simulink model "AynchronousEKF_SimpleCircleTrajectory"  (R2025b)
settings: Solver=VariableStepAuto  StartTime=0.0  StopTime=100  RelTol=1e-3
undefined symbols (not defined in the file or in its folder): cam1_sample_time, cam2_sample_time, cam3_sample_time, cam_intrinsics, dt_ekf, focusLength_narrow, gray, num_cams, omega, pixelSize, radius, Rec, resolution, SDTV, Sim3dSensor, waypointTrajectory
libraries: sim3dlib x10, robotcorelib x7, visionconversions x6, sim3dcameralib x3, uavutilslib x1, uavsim3dlib x1, uavalgslib x1, dspnetwork x1
settings Model: Creator=nnekoo  LastModifiedBy=Shannon Pitman

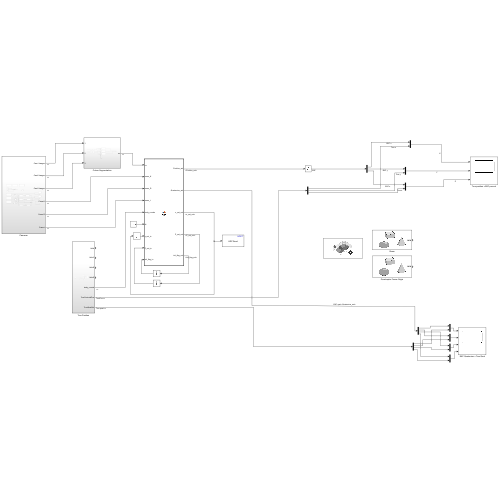
[thumbnail: Simulink's stored preview of the top-level diagram]
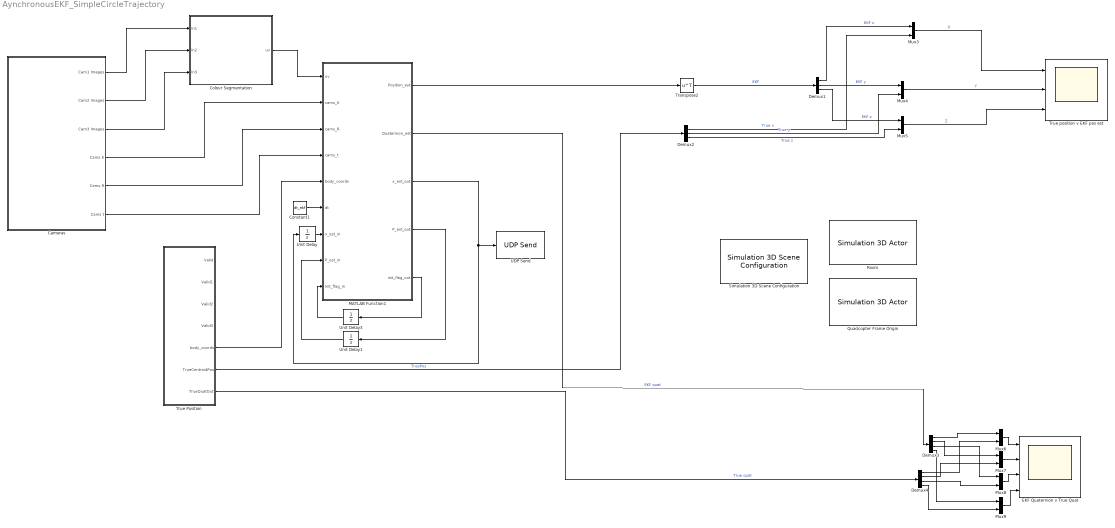
== system AynchronousEKF_SimpleCircleTrajectory ==
  " EKF Quaternion v True Quat" : Scope  NumInputPorts=4
      settings: ActiveDisplayYMinimum=-1.2499889931974075  ActiveDisplayYMaximum=1.2499985502233475  DataLoggingVariableName=ScopeData2
  Cameras : Subsystem
  Colour Segmentation : Subsystem
  Constant1 : Constant  Value=dt_ekf
  Demux1 : Demux  Outputs=3
  Demux2 : Demux  Outputs=3
  Demux3 : Demux
  Demux4 : Demux
  MATLAB Function1 : MATLAB Function  TreatAsAtomicUnit=on
  Mux{3..9} (7 alike) : Mux  Inputs=2
  Quadcopter Frame Origin : sim3dlib/Simulation 3D Actor  Priority=1  ActorName=QuadcopterOrigin  ParentName=Quadcopter  Operation=Create at setup  InitScriptText=|  SampleTime=-1  Translation=[0 0 0]  Rotation=[0 0 0]  Scale=[.01 .01 .01]  aMode=aMode  ActorTag=QuadcopterOrigin  ActorType=Sim3dActor  ID=C
      | createShape(Actor, 'cylinder', [1 1 1]);
      | 
      | Actor.Color = [255 192 203]/255;
      | Actor.Mobility = sim3d.utils.MobilityTypes.Movable;
  Room : sim3dlib/Simulation 3D Actor  Priority=1  ActorName=Room  ParentName=Scene Origin  Operation=Create at setup  InitScriptText=|  SampleTime=-1  Translation=[0 0 0]  Rotation=[0 0 0]  Scale=[1 1 1]  aMode=5  ActorTag=Room  ActorType=Sim3dActor  ID=C
      | leftWall = sim3d.Actor(ActorName="leftWall");
      | createShape(leftWall, 'plane', [8 5 1]);
      | leftWall.Rotation = [pi/2 0 0];
      | leftWall.Translation = [0 -4.5 1.5];
      | leftWall.Color = [1 1 1];
      | World.add(leftWall,Actor);
      | 
      | rightWall = sim3d.Actor(ActorName="rightWall");
      | createShape(rightWall, 'plane', [8 5 1]);
      | % rightWall.CoordinateSystem = 'MATLAB';
      | rightWall.Rotation = [pi/2 0 0];
      | rightWall.Translation = [0 4.5 1.5];
      | rightWall.Color = [1 1 1];
      | World.add(rightWall,Actor);
      | 
      | farWall = sim3d.Actor(ActorName="farWall");
      | createShape(farWall, 'plane', [9 5 1]);
      | % farWall.CoordinateSystem = 'MATLAB';
      | farWall.Rotation = [pi/2 0 pi/2];
      | farWall.Translation = [4 0 1.5];
      | farWall.TwoSided = true;
      | farWall.Color = [1 1 1];
      | World.add(farWall,Actor);
      | 
      | floor = sim3d.Actor(ActorName="floor");
      | createShape(floor, 'plane', [8 9 .5]);
      | % floor.CoordinateSystem = 'MATLAB';
      | floor.Translation = [0 0 -1];
      | floor.Rotation = [0 0 0];
      | floor.Color = [1 1 1];
      | World.add(floor,Actor);
      | 
      | ceiling = sim3d.Actor(ActorName="ceiling");
      | createShape(ceiling, 'plane', [8 9 .5]);
      | % floor.CoordinateSystem = 'MATLAB';
      | ceiling.Translation = [0 0 4];
      | ceiling.Rotation = [0 0 0];
      | ceiling.Color = [1 1 1];
      | World.add(ceiling,Actor);
      | 
      | frontWall = sim3d.Actor(ActorName="frontWall");
      | createShape(frontWall, 'plane', [9 5 1]);
      | % floor.CoordinateSystem = 'MATLAB';
      | frontWall.Rotation = [pi/2 0 pi/2];
      | frontWall.Translation = [-4 0 1.5];
      | World.add(frontWall,Actor);
      | 
      | lights = sim3d.Light(ActorName = 'ceilingLights', NumberOfLights=7, LightType = 'PointLight', Translation = [-3 -3 3.9; 3 -3 3.9;0 -3 3.9; 0 3 3.9; -3 3 3.9;3 3 3.9; 0 0 3.9 ]);
      | World.add(lights, Actor);
      | %, Rotation = [pi/2 0 pi/2; pi/2 0 pi/2; pi/2 0 pi/2; pi/2 0 pi/2]
  Simulation 3D Scene Configuration : sim3dlib/Simulation 3D Scene Configuration  Priority=0  ProjectFormat=Default Scenes  SceneDesc=Empty scene  ProjectName=C:\Program Files\MATLAB\R2025b\toolbox\shared\sim3d_projects\automotive_project_windows\UE\WindowsNoEditor\VehicleSimulation.exe  ScenePath=/Game/Maps/HwStrght  UEProjPath=C:\project\AutoVrtlEnv\AutoVrtlEnv.uproject  EnableOpenDRIVE=off  vehTagList={'Cam1';'Cam2';'Cam3';'Custom';'FrontLeftMotor';'FrontRightMotor';'Quadcopter';'QuadcopterOrigin';'RearLeftMotor';'RearRightMotor';'Room';'Scene Origin'}  vehTag=Custom  AttachedCameraRelativeTranslation=[0 0 0]  FreeCameraDefaultInitialTranslation=[-6, 0, 2]  AttachedCameraRelativeRotation=[0 0 0]  FreeCameraDefaultInitialRotation=[0, -15, 0]  ViewpointName=Custom  FreeCameraInitialTranslation=[-3 0 0.5]  ViewpointTranslation=[0 0 0]  FreeCameraInitialRotation=[0 -10 0]  ViewpointRotation=[0 0 0]  OpVisEn=off  Ts=1/60  EnableWindow=off  EnableRemoteAccess=off  EnableWeather=off  SunAzimuth=90  SunAltitude=40.0  EnableGeospatialSun=off  Latitude=0  Longitude=0  Date=2023-01-01  Time=10:30:00  GeoTimeZone=-5.0  SunDaylightSaving=off  wind=1  clouds=10  EnableVolumetricClouds=off  CloudCoverage=0  CloudAltitude=6  fog=0  rain=0  RaindropsEffect=off  SnowDensity=0  EnableGeospatial=off  TilesetSource=Earth terrain  UseTrueOrigin=off  OriginHeight=200  OriginLatitude=40.744652  OriginLongitude=-73.988864  MapStyle=Aerial  AdditionalAssetIDs=[]  UseAdvancedSunSky=off  SolarTime=11  TimeZone=-5  Day=21  Month=9  Year=2022  UseDaylightSavingTime=on  DSTStartDay=10  DSTStartMonth=3  DSTEndDay=3  DSTEndMonth=11  DSTSwitchHour=2  sensorTag=MainCamera1  sensorId=1  sensorName=MainCamera1  mountLoc=Origin  offsetFlag=off  tmountOffset=[0, 0, 0]  rmountOffset=[0, 0, 0]  HorizontalResolution=1280  VerticalResolution=720  HorizontalFOV=60  mountPoint=[0 0 0]  mountOrientation=[0 0 0]  aMode=5  ID=1  GeoTrigger=Inactive  ViewNameList={'Custom'}  ViewTranslationList={'[-3 0 0.5]'}  ViewRotationList={'[0 -10 0]'}
      settings: LibrarySourceBlock=sl3dlib/Simulation 3D/Environment/Simulation 3D Scene Configuration
  Transpose2 : Math  Operator=transpose
  True Position : Subsystem
  True position v EKF pos est : Scope  NumInputPorts=3
      settings: ActiveDisplayYMinimum=1.2433440169653658  ActiveDisplayYMaximum=2.8099234426996063
  UDP Send : dspnetwork/UDP Send  remoteURL='127.0.0.1'  remotePort=25000  localURL='0.0.0.0'  localPortSource=Automatically determine  localPort=-1  sendBufferSize=8192  sampletime=-1  blockPlatform=HOST  separateLengthPort=0
      settings: LibrarySourceBlock=embeddedtargetslib/Host Communication/UDP Send
  Unit Delay : UnitDelay  InitialCondition=zeros(13,1)  SampleTime=dt_ekf  StateName=Previous State Estimate  HasFrameUpgradeWarning=on
  Unit Delay1 : UnitDelay  InitialCondition=zeros(13,13)  SampleTime=dt_ekf  StateName=Previous State Error Covariance Estimate  HasFrameUpgradeWarning=on
  Unit Delay3 : UnitDelay  SampleTime=dt_ekf  StateName=EKF has been initialised  HasFrameUpgradeWarning=on
  wires:
  MATLAB Function1/1(Position_est) -> Transpose2/1
  Constant1/1 -> MATLAB Function1/6(dt)
  True Position/5(body_coords) -> MATLAB Function1/5(body_coords)
  MATLAB Function1/2(Quaternion_est) -> Demux3/1  "EKF quat"
  MATLAB Function1/3(x_est_out) -> UDP Send/1, Unit Delay/1
  Unit Delay/1 -> MATLAB Function1/7(x_est_in)
  Unit Delay1/1 -> MATLAB Function1/8(P_est_in)
  Unit Delay3/1 -> MATLAB Function1/9(init_flag_in)
  Transpose2/1 -> Demux1/1  "EKF"
  Demux1/1 -> Mux3/1  "EKF x"
  Demux2/1 -> Mux3/2  "True x"
  Demux1/2 -> Mux4/1  "EKF y"
  Demux2/2 -> Mux4/2  "True y"
  Demux1/3 -> Mux5/1  "EKF z"
  Mux3/1 -> True position v EKF pos est/1  "X"
  Demux2/3 -> Mux5/2  "True z"
  Mux4/1 -> True position v EKF pos est/2  "Y"
  Mux5/1 -> True position v EKF pos est/3  "Z"
  Demux3/1 -> Mux6/1
  Demux4/1 -> Mux6/2
  Mux6/1 -> " EKF Quaternion v True Quat"/1
  Demux3/2 -> Mux7/1
  Demux4/2 -> Mux7/2
  Mux7/1 -> " EKF Quaternion v True Quat"/2
  Demux3/3 -> Mux8/1
  Demux4/3 -> Mux8/2
  Mux8/1 -> " EKF Quaternion v True Quat"/3
  Demux3/4 -> Mux9/1
  Demux4/4 -> Mux9/2
  Mux9/1 -> " EKF Quaternion v True Quat"/4
  True Position/6(TrueCentroidPos) -> Demux2/1  "TruePos"
  True Position/7(TrueQuatOut) -> Demux4/1  "True quat"
  Cameras/1(Cam1 Images) -> Colour Segmentation/1(In1)
  Cameras/2(Cam2 Images) -> Colour Segmentation/2(In2)
  Cameras/3(Cam3 Images) -> Colour Segmentation/3(In3)
  Cameras/4(Cams.K) -> MATLAB Function1/2(cams_K)
  Cameras/5(Cams.R) -> MATLAB Function1/3(cams_R)
  Cameras/6(Cams.t) -> MATLAB Function1/4(cams_t)
  Colour Segmentation/1(uv) -> MATLAB Function1/1(uv)
  MATLAB Function1/5(init_flag_out) -> Unit Delay3/1
  MATLAB Function1/4(P_est_out) -> Unit Delay1/1

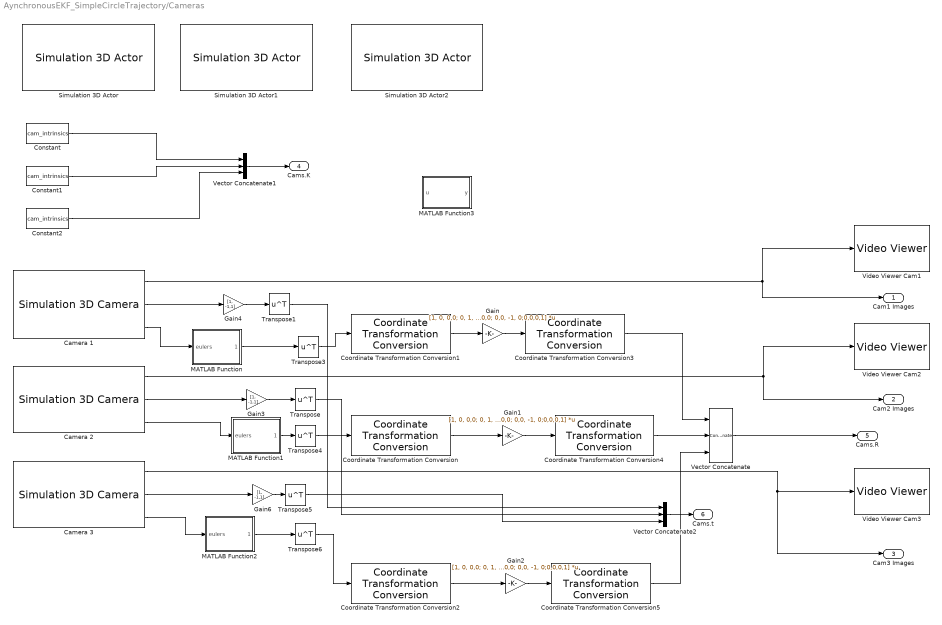
== system AynchronousEKF_SimpleCircleTrajectory/Cameras ==
  Camera 1 : sim3dcameralib/Simulation 3D Camera  Priority=1  sensorTag=Sim3dSensor�  sensorId=1  sensorName=Sim3dSensor�  vehTagList={'Cam1';'Cam2';'Cam3';'FrontLeftMotor';'FrontRightMotor';'Quadcopter';'QuadcopterOrigin';'RearLeftMotor';'RearRightMotor';'Room';'Scene Origin'}  vehTag=Scene Origin  CoordinateSystem=Default  mountLoc=Origin  offsetFlag=on  tmountOffset=[0, -2, 0.5]  extTmount=off  rmountOffset=[0, 0, pi/4]  extRmount=off  FocalLength=[focusLength_narrow/pixelSize(1), focusLength_narrow/pixelSize(2)]  OpticalCenter=[resolution(2)/2 resolution(1)/2]  ImageSize=resolution  RadialDistortion=[0, 0]  TangentialDistortion=[0, 0]  SensorSkew=0  VisualizeFieldOfView=off  FieldOfViewRange=61  DepthOutportEnabled=off  SemanticOutportEnabled=off  TransformOutportEnabled=on  SampleTime=cam1_sample_time  mountPoint=[0 -2 0.5]  mountOrientation=[0 0 0.785398163397448]  aMode=5  ID=1
      settings: LibrarySourceBlock=sl3dlib/Simulation 3D/Sensors/Simulation 3D Camera
  Camera 2 : sim3dcameralib/Simulation 3D Camera  Priority=1  sensorTag=Sim3dSensor�  sensorId=2  sensorName=Sim3dSensor�  vehTagList={'Cam1';'Cam2';'Cam3';'FrontLeftMotor';'FrontRightMotor';'Quadcopter';'QuadcopterOrigin';'RearLeftMotor';'RearRightMotor';'Room';'Scene Origin'}  vehTag=Scene Origin  CoordinateSystem=Default  mountLoc=Origin  offsetFlag=on  tmountOffset=[0, 2, 0.5]  extTmount=off  rmountOffset=[0, 0, -pi/4]  extRmount=off  FocalLength=[focusLength_narrow/pixelSize(1), focusLength_narrow/pixelSize(2)]  OpticalCenter=[resolution(2)/2 resolution(1)/2]  ImageSize=resolution  RadialDistortion=[0, 0]  TangentialDistortion=[0, 0]  SensorSkew=0  VisualizeFieldOfView=off  FieldOfViewRange=61  DepthOutportEnabled=off  SemanticOutportEnabled=off  TransformOutportEnabled=on  SampleTime=cam2_sample_time  mountPoint=[0 2 0.5]  mountOrientation=[0 0 -0.785398163397448]  aMode=5  ID=2
      settings: LibrarySourceBlock=sl3dlib/Simulation 3D/Sensors/Simulation 3D Camera
  Camera 3 : sim3dcameralib/Simulation 3D Camera  Priority=1  sensorTag=Sim3dSensor�  sensorId=3  sensorName=Sim3dSensor�  vehTagList={'Cam1';'Cam2';'Cam3';'FrontLeftMotor';'FrontRightMotor';'Quadcopter';'QuadcopterOrigin';'RearLeftMotor';'RearRightMotor';'Room';'Scene Origin'}  vehTag=Scene Origin  CoordinateSystem=Default  mountLoc=Origin  offsetFlag=on  tmountOffset=[2.5,-1.5,0.5]  extTmount=off  rmountOffset=[0, 0, pi/2]  extRmount=off  FocalLength=[focusLength_narrow/pixelSize(1), focusLength_narrow/pixelSize(2)]  OpticalCenter=[resolution(2)/2 resolution(1)/2]  ImageSize=resolution  RadialDistortion=[0, 0]  TangentialDistortion=[0, 0]  SensorSkew=0  VisualizeFieldOfView=off  FieldOfViewRange=61  DepthOutportEnabled=off  SemanticOutportEnabled=off  TransformOutportEnabled=on  SampleTime=cam3_sample_time  mountPoint=[2.5 -1.5 0.5]  mountOrientation=[0 0 1.5707963267949]  aMode=5  ID=3
      settings: LibrarySourceBlock=sl3dlib/Simulation 3D/Sensors/Simulation 3D Camera
  Constant : Constant  Value=cam_intrinsics  VectorParams1D=off
  Constant1 : Constant  Value=cam_intrinsics  VectorParams1D=off
  Constant2 : Constant  Value=cam_intrinsics  VectorParams1D=off
  Coordinate Transformation Conversion : robotcorelib/Coordinate Transformation Conversion  InputRepresentation=Euler Angles  InputEulerSequence=ZYX  ShowTrVecInputPort=on  OutputRepresentation=Quaternion  OutputEulerSequence=ZYX  ShowTrVecOutputPort=on  SimulateUsing=Interpreted execution
      settings: LibrarySourceBlock=navlib/Utilities/Coordinate Transformation Conversion
  Coordinate Transformation Conversion1 : robotcorelib/Coordinate Transformation Conversion  InputRepresentation=Euler Angles  InputEulerSequence=ZYX  ShowTrVecInputPort=on  OutputRepresentation=Quaternion  OutputEulerSequence=ZYX  ShowTrVecOutputPort=on  SimulateUsing=Interpreted execution
      settings: LibrarySourceBlock=navlib/Utilities/Coordinate Transformation Conversion
  Coordinate Transformation Conversion2 : robotcorelib/Coordinate Transformation Conversion  InputRepresentation=Euler Angles  InputEulerSequence=ZYX  ShowTrVecInputPort=on  OutputRepresentation=Quaternion  OutputEulerSequence=ZYX  ShowTrVecOutputPort=on  SimulateUsing=Interpreted execution
      settings: LibrarySourceBlock=navlib/Utilities/Coordinate Transformation Conversion
  Coordinate Transformation Conversion3 : robotcorelib/Coordinate Transformation Conversion  InputRepresentation=Quaternion  InputEulerSequence=XYZ  ShowTrVecInputPort=on  OutputRepresentation=Rotation Matrix  OutputEulerSequence=ZYX  ShowTrVecOutputPort=on  SimulateUsing=Interpreted execution
      settings: LibrarySourceBlock=navlib/Utilities/Coordinate Transformation Conversion
  Coordinate Transformation Conversion4 : robotcorelib/Coordinate Transformation Conversion  InputRepresentation=Quaternion  InputEulerSequence=XYZ  ShowTrVecInputPort=on  OutputRepresentation=Rotation Matrix  OutputEulerSequence=ZYX  ShowTrVecOutputPort=on  SimulateUsing=Interpreted execution
      settings: LibrarySourceBlock=navlib/Utilities/Coordinate Transformation Conversion
  Coordinate Transformation Conversion5 : robotcorelib/Coordinate Transformation Conversion  InputRepresentation=Quaternion  InputEulerSequence=XYZ  ShowTrVecInputPort=on  OutputRepresentation=Rotation Matrix  OutputEulerSequence=ZYX  ShowTrVecOutputPort=on  SimulateUsing=Interpreted execution
      settings: LibrarySourceBlock=navlib/Utilities/Coordinate Transformation Conversion
  Gain : Gain  Gain=[1, 0, 0,0; 0, 1, 0,0; 0,0, -1, 0;0,0,0,1]  Multiplication=Matrix(K*u)
  Gain1 : Gain  Gain=[1, 0, 0,0; 0, 1, 0,0; 0,0, -1, 0;0,0,0,1]  Multiplication=Matrix(K*u)
  Gain2 : Gain  Gain=[1, 0, 0,0; 0, 1, 0,0; 0,0, -1, 0;0,0,0,1]  Multiplication=Matrix(K*u)
  Gain3 : Gain  Gain=[1, -1,1]
  Gain4 : Gain  Gain=[1, -1,1]
  Gain6 : Gain  Gain=[1, -1,1]
  MATLAB Function : MATLAB Function  TreatAsAtomicUnit=on
  MATLAB Function1 : MATLAB Function  TreatAsAtomicUnit=on
  MATLAB Function2 : MATLAB Function  TreatAsAtomicUnit=on
  MATLAB Function3 : MATLAB Function  TreatAsAtomicUnit=on
  Simulation 3D Actor : sim3dlib/Simulation 3D Actor  Priority=1  ActorName=Cam1  ParentName=Camera1  Operation=Create at setup  InitScriptText=|  SampleTime=-1  Translation=[0 0 0]  Rotation=[0 0 0]  Scale=[1 1 1]  aMode=5  ActorTag=Cam1  ActorType=Sim3dActor  ID=C
      | createShape(Actor, 'cylinder', [0.1 0.1 0.1]);
      | 
      | % Initialize values (optional)
      | Actor.Color = [0 0 0];
      | Actor.CoordinateSystem = 'MATLAB';
      | 
      | % Reserved keywords:
      | % - Actor : handle to this actor object
      | % - World : handle to the world object
      | 
      | % Examples:
      | 
      | % Create a primitive geometry (optional)
      | % createShape(Actor, 'box', [1 1 1]);
      | 
      | % Initialize values (optional)
      | % Actor.Physics = true;
      | % Actor.Color = [1 0 0];
  Simulation 3D Actor1 : sim3dlib/Simulation 3D Actor  Priority=1  ActorName=Cam2  ParentName=Camera2  Operation=Create at setup  InitScriptText=|  SampleTime=-1  Translation=[0 0 0]  Rotation=[0 0 0]  Scale=[1 1 1]  aMode=5  ActorTag=Cam2  ActorType=Sim3dActor  ID=C
      | createShape(Actor, 'cylinder', [0.1 0.1 0.1]);
      | 
      | % Initialize values (optional)
      | Actor.Color = [1 0.65 0];
      | Actor.CoordinateSystem = 'MATLAB';
      | % Reserved keywords:
      | % - Actor : handle to this actor object
      | % - World : handle to the world object
      | 
      | % Examples:
      | 
      | % Create a primitive geometry (optional)
      | % createShape(Actor, 'box', [1 1 1]);
      | 
      | % Initialize values (optional)
      | % Actor.Physics = true;
      | % Actor.Color = [1 0 0];
  Simulation 3D Actor2 : sim3dlib/Simulation 3D Actor  Priority=1  ActorName=Cam3  ParentName=Camera3  Operation=Create at setup  InitScriptText=|  SampleTime=-1  Translation=[0 0 0]  Rotation=[0 0 0]  Scale=[1 1 1]  aMode=5  ActorTag=Cam3  ActorType=Sim3dActor  ID=C
      | createShape(Actor, 'cylinder', [0.1 0.1 0.1]);
      | 
      | % Initialize values (optional)
      | Actor.Color = [1 1 1];
      | Actor.CoordinateSystem = 'MATLAB';
      | % Reserved keywords:
      | % - Actor : handle to this actor object
      | % - World : handle to the world object
      | 
      | % Examples:
      | 
      | % Create a primitive geometry (optional)
      | % createShape(Actor, 'box', [1 1 1]);
      | 
      | % Initialize values (optional)
      | % Actor.Physics = true;
      | % Actor.Color = [1 0 0];
  Transpose{,1,3..6} (6 alike) : Math  Operator=transpose
  Vector Concatenate : Concatenate  NumInputs=3  Mode=Multidimensional array
  Vector Concatenate1 : Concatenate  NumInputs=3  Mode=Multidimensional array
  Vector Concatenate2 : Concatenate  NumInputs=3
  Video Viewer Cam1 : VideoViewer  colormapValue=gray(256)  FigPos=[-793 733 418 262]
  Video Viewer Cam2 : VideoViewer  colormapValue=gray(256)  FigPos=[-1221 623 418 282]
  Video Viewer Cam3 : VideoViewer  colormapValue=gray(256)  FigPos=[-1491 936 417 301]
  Cam1 Images : Outport
  Cam2 Images : Outport  Port=2
  Cam3 Images : Outport  Port=3
  Cams.K : Outport  Port=4
  Cams.R : Outport  Port=5
  Cams.t : Outport  Port=6
  wires:
  Transpose3/1 -> Coordinate Transformation Conversion1/1
  Transpose6/1 -> Coordinate Transformation Conversion2/1
  Transpose4/1 -> Coordinate Transformation Conversion/1
  Constant/1 -> Vector Concatenate1/1
  Constant1/1 -> Vector Concatenate1/2
  Constant2/1 -> Vector Concatenate1/3
  Vector Concatenate/1 -> Cams.R/1
  Vector Concatenate1/1 -> Cams.K/1
  Vector Concatenate2/1 -> Cams.t/1
  Camera 3/2 -> Gain6/1
  Camera 2/2 -> Gain3/1
  Camera 1/2 -> Gain4/1
  Coordinate Transformation Conversion1/1 -> Gain/1
  Coordinate Transformation Conversion/1 -> Gain1/1
  Coordinate Transformation Conversion2/1 -> Gain2/1
  Transpose1/1 -> Vector Concatenate2/1
  Transpose/1 -> Vector Concatenate2/2
  Transpose5/1 -> Vector Concatenate2/3
  Gain6/1 -> Transpose5/1
  Gain3/1 -> Transpose/1
  Gain4/1 -> Transpose1/1
  Camera 2/3 -> MATLAB Function1/1(eulers)
  Camera 3/3 -> MATLAB Function2/1(eulers)
  Camera 1/3 -> MATLAB Function/1(eulers)
  Gain/1 -> Coordinate Transformation Conversion3/1
  Coordinate Transformation Conversion3/1 -> Vector Concatenate/1
  Gain1/1 -> Coordinate Transformation Conversion4/1
  Coordinate Transformation Conversion4/1 -> Vector Concatenate/2
  Gain2/1 -> Coordinate Transformation Conversion5/1
  Coordinate Transformation Conversion5/1 -> Vector Concatenate/3
  MATLAB Function/1(eulerZYX) -> Transpose3/1
  MATLAB Function1/1(eulerZYX) -> Transpose4/1
  MATLAB Function2/1(eulerZYX) -> Transpose6/1
  Camera 1/1 -> Cam1 Images/1, Video Viewer Cam1/1
  Camera 2/1 -> Cam2 Images/1, Video Viewer Cam2/1
  Camera 3/1 -> Cam3 Images/1, Video Viewer Cam3/1

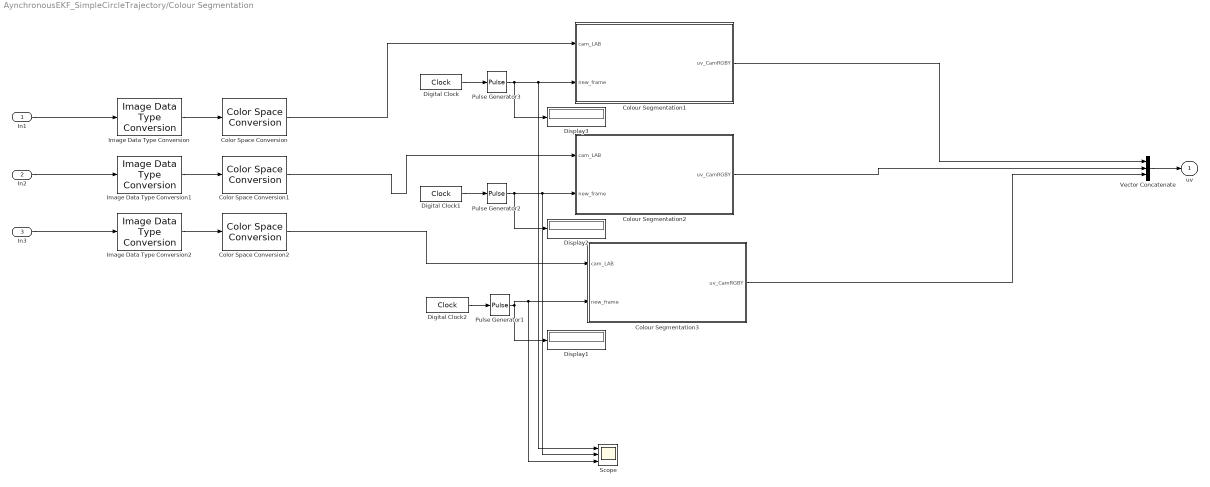
== system AynchronousEKF_SimpleCircleTrajectory/Colour Segmentation ==
  In1 : Inport
  In2 : Inport  Port=2
  In3 : Inport  Port=3
  Color Space Conversion : visionconversions/Color Space  Conversion  conversion=Obsolete  conversionActive=sR'G'B' to L*a*b*  wp_str=D65  rec=Rec. 601 (SDTV)  sys=1125/60/2:1  imagePorts=One multidimensional signal
  Color Space Conversion1 : visionconversions/Color Space  Conversion  conversion=Obsolete  conversionActive=sR'G'B' to L*a*b*  wp_str=D65  rec=Rec. 601 (SDTV)  sys=1125/60/2:1  imagePorts=One multidimensional signal
  Color Space Conversion2 : visionconversions/Color Space  Conversion  conversion=Obsolete  conversionActive=sR'G'B' to L*a*b*  wp_str=D65  rec=Rec. 601 (SDTV)  sys=1125/60/2:1  imagePorts=One multidimensional signal
  Colour Segmentation1 : MATLAB Function  TreatAsAtomicUnit=on
  Colour Segmentation2 : MATLAB Function  TreatAsAtomicUnit=on
  Colour Segmentation3 : MATLAB Function  TreatAsAtomicUnit=on
  Digital Clock : DigitalClock  SampleTime=cam1_sample_time/num_cams
  Digital Clock1 : DigitalClock  SampleTime=cam2_sample_time/num_cams
  Digital Clock2 : DigitalClock  SampleTime=cam3_sample_time/num_cams
  Display1 : Display
  Display2 : Display
  Display3 : Display
  Image Data Type Conversion : visionconversions/Image Data Type Conversion  outDT=double  isSigned=on  wordLen=16  numFracBits=0
  Image Data Type Conversion1 : visionconversions/Image Data Type Conversion  outDT=double  isSigned=on  wordLen=16  numFracBits=0
  Image Data Type Conversion2 : visionconversions/Image Data Type Conversion  outDT=double  isSigned=on  wordLen=16  numFracBits=0
  Pulse Generator1 : DiscretePulseGenerator  TimeSource=Use external signal  Period=3  PhaseDelay=2  SampleTime=1/60
  Pulse Generator2 : DiscretePulseGenerator  TimeSource=Use external signal  Period=3  PhaseDelay=1  SampleTime=1/60
  Pulse Generator3 : DiscretePulseGenerator  TimeSource=Use external signal  Period=3  SampleTime=1/60
  Scope : Scope  NumInputPorts=3
      settings: ActiveDisplayYMinimum=-0.036926070641322362  ActiveDisplayYMaximum=1.1105177004394333
  Vector Concatenate : Concatenate  NumInputs=3  Mode=Multidimensional array
  uv : Outport
  wires:
  Image Data Type Conversion/1 -> Color Space Conversion/1
  Image Data Type Conversion1/1 -> Color Space Conversion1/1
  Colour Segmentation1/1(uv_CamRGBY) -> Vector Concatenate/1
  Colour Segmentation2/1(uv_CamRGBY) -> Vector Concatenate/2
  Color Space Conversion1/1 -> Colour Segmentation2/1(cam_LAB)
  In1/1 -> Image Data Type Conversion/1
  In2/1 -> Image Data Type Conversion1/1
  In3/1 -> Image Data Type Conversion2/1
  Image Data Type Conversion2/1 -> Color Space Conversion2/1
  Vector Concatenate/1 -> uv/1
  Colour Segmentation3/1(uv_CamRGBY) -> Vector Concatenate/3
  Pulse Generator3/1 -> Display3/1, Scope/1, Colour Segmentation1/2(new_frame)
  Color Space Conversion2/1 -> Colour Segmentation3/1(cam_LAB)
  Color Space Conversion/1 -> Colour Segmentation1/1(cam_LAB)
  Digital Clock/1 -> Pulse Generator3/1
  Digital Clock1/1 -> Pulse Generator2/1
  Pulse Generator2/1 -> Scope/2, Colour Segmentation2/2(new_frame), Display2/1
  Digital Clock2/1 -> Pulse Generator1/1
  Pulse Generator1/1 -> Colour Segmentation3/2(new_frame), Scope/3, Display1/1

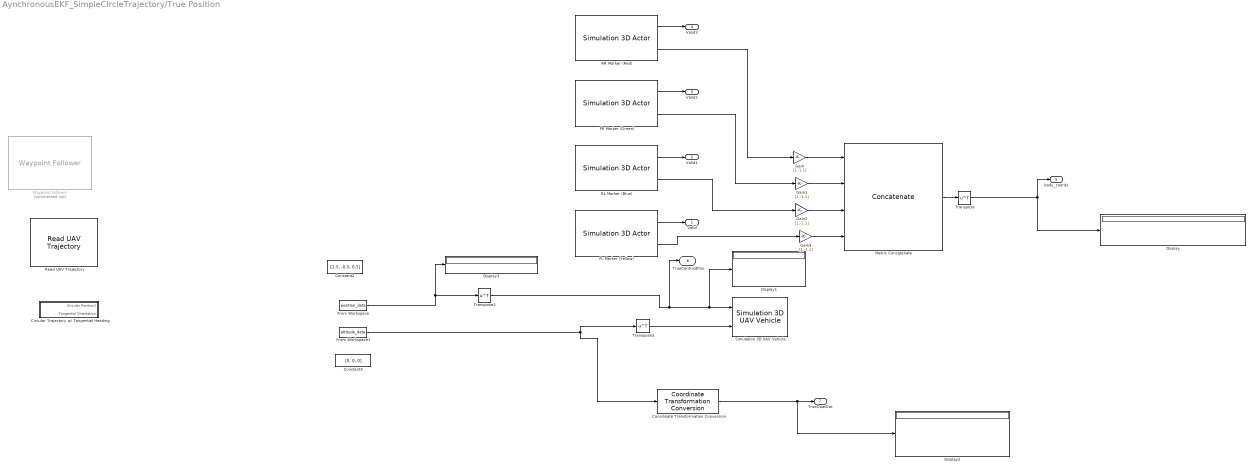
== system AynchronousEKF_SimpleCircleTrajectory/True Position ==
  Circular Trajectory w/ Tangential Heading : Subsystem
  Constant2 : Constant  Value=[2.5, -0.5, 0.5]  VectorParams1D=off
  Constant3 : Constant  Value=[0, 0, 0]  VectorParams1D=off
  Coordinate Transformation Conversion : robotcorelib/Coordinate Transformation Conversion  InputRepresentation=Euler Angles  InputEulerSequence=ZYX  ShowTrVecInputPort=on  OutputRepresentation=Quaternion  OutputEulerSequence=ZYX  ShowTrVecOutputPort=on  SimulateUsing=Interpreted execution
      settings: LibrarySourceBlock=navlib/Utilities/Coordinate Transformation Conversion
  Display{,1..3} (4 alike) : Display
  FL Marker (Yellow) : sim3dlib/Simulation 3D Actor  Priority=1  ActorName=FrontLeftMotor  ParentName=Quadcopter  Operation=Create at setup  InitScriptText=|  SampleTime=-1  Translation=[0.134 -0.137 0.192]  Rotation=[0 9 48.32-90]/180*pi  Scale=[.035 .035 .03]  OutputsText=FrontLeftMotor.Translation  aMode=aMode  ActorTag=FrontLeftMotor  ActorType=Sim3dActor  ID=C
      | createShape(Actor, 'cylinder', [1 1 1]);
      | 
      | % Initialize values (optional)
      | Actor.Color = [1 1 0];
      | Actor.Shininess = 0.1;
      | Actor.Mobility = sim3d.utils.MobilityTypes.Movable;
  FR Marker (Green) : sim3dlib/Simulation 3D Actor  Priority=1  ActorName=FrontRightMotor  ParentName=Quadcopter  Operation=Create at setup  InitScriptText=|  SampleTime=-1  Translation=[0.134 0.137 0.192]  Rotation=[0 9 48.32]/180*pi  Scale=[.035 .035 .03]  OutputsText=FrontRightMotor.Translation  aMode=aMode  ActorTag=FrontRightMotor  ActorType=Sim3dActor  ID=C
      | createShape(Actor, 'cylinder', [1 1 1]);
      | 
      | % Initialize values (optional)
      | Actor.Color = [0 1 0];
      | Actor.Shininess = 0.1;
      | Actor.Mobility = sim3d.utils.MobilityTypes.Movable;
  From Workspace : FromWorkspace  VariableName=position_data  SampleTime=1/60
  From Workspace1 : FromWorkspace  VariableName=attitude_data  SampleTime=1/60
  Gain{,1..3} (4 alike) : Gain  Gain=[1,-1,1]
  Matrix Concatenate : Concatenate  NumInputs=4  Mode=Multidimensional array
  RL Marker (Blue) : sim3dlib/Simulation 3D Actor  Priority=1  ActorName=RearLeftMotor  ParentName=Quadcopter  Operation=Create at setup  InitScriptText=|  SampleTime=-1  Translation=[-0.134 -0.137 0.192]  Rotation=[0 9 48.32-180]/180*pi  Scale=[.035 .035 .03]  OutputsText=RearLeftMotor.Translation  aMode=aMode  ActorTag=RearLeftMotor  ActorType=Sim3dActor  ID=C
      | createShape(Actor, 'cylinder', [1 1 1]);
      | 
      | % Initialize values (optional)
      | Actor.Color = [0.08 0.18 1];
      | Actor.Shininess = 0.1;
      | Actor.Mobility = sim3d.utils.MobilityTypes.Movable;
  RR Marker (Red) : sim3dlib/Simulation 3D Actor  Priority=1  ActorName=RearRightMotor  ParentName=Quadcopter  Operation=Create at setup  InitScriptText=|  SampleTime=-1  Translation=[-0.134 0.137 0.192]  Rotation=[0 9 48.32+90]/180*pi  Scale=[.035 .035 .03]  OutputsText=RearRightMotor.Translation  aMode=aMode  ActorTag=RearRightMotor  ActorType=Sim3dActor  ID=C
      | createShape(Actor, 'cylinder', [1 1 1]);
      | 
      | % Initialize values (optional)
      | Actor.Color = [1 0 0];
      | Actor.Shininess = 0.1;
      | Actor.Mobility = sim3d.utils.MobilityTypes.Movable;
  Read UAV Trajectory : uavutilslib/Read UAV Trajectory  TrajectorySource=From trajectory object in workspace  ScenarioObj=singleUAVScenario  PlatformName=UAV  TrajectoryObj=waypointTrajectory()  TransformToENU=on  FrameConversionDisplay=NED → ENU
  Simulation 3D UAV Vehicle : uavsim3dlib/Simulation 3D UAV Vehicle  Priority=-1  Mesh=Quadrotor  MeshPath=/MathWorksUAVContent/UAVs/HexaRotorUAV/HexaRotor.HexaRotor  Color=Black  ActorName=Quadcopter  UseGlobalFrame=off  InitialTranslation=[2.6 0 0.5]  InitialRotation="[1.5708  0 0]"  InitialTranslationGlobal=[0 0 0]  InitialGeoOrigin=[0 0 0]  InitialRotationGlobal=[0 0 0]  SampleTime=-1  ActorType=SimulinkVehicle  ID=C  aMode=4  ActorTag=Quadcopter
  Transpose : Math  Operator=transpose
  Transpose2 : Math  Operator=transpose
  Transpose3 : Math  Operator=transpose
  Waypoint Follower : uavalgslib/Waypoint Follower  Commented=on  UAVType=multirotor  StartFrom=first  TransitionRadiusSource=internal  TransitionRadius=10  MinLookaheadDistance=0.1  HoverAtLastWaypoint=off  YawInput=off  ShowCrossTrackErrorOutput=off  ShowStatusOutput=off  SimulateUsing=Interpreted execution
  Valid : Outport
  Valid1 : Outport  Port=2
  Valid2 : Outport  Port=3
  Valid3 : Outport  Port=4
  body_coords : Outport  Port=5
  TrueCentroidPos : Outport  Port=6
  TrueQuatOut : Outport  Port=7
  wires:
  RL Marker (Blue)/1 -> Valid1/1
  RR Marker (Red)/1 -> Valid3/1
  FR Marker (Green)/1 -> Valid2/1
  FL Marker (Yellow)/1 -> Valid/1
  Matrix Concatenate/1 -> Transpose/1
  Coordinate Transformation Conversion/1 -> TrueQuatOut/1, Display2/1
  Transpose/1 -> Display/1, body_coords/1
  From Workspace/1 -> Transpose2/1, Display3/1
  From Workspace1/1 -> Coordinate Transformation Conversion/1, Transpose3/1
  RR Marker (Red)/2 -> Gain/1
  FR Marker (Green)/2 -> Gain1/1
  RL Marker (Blue)/2 -> Gain2/1
  FL Marker (Yellow)/2 -> Gain3/1
  Gain/1 -> Matrix Concatenate/1
  Gain1/1 -> Matrix Concatenate/2
  Gain2/1 -> Matrix Concatenate/3
  Gain3/1 -> Matrix Concatenate/4
  Transpose2/1 -> Display1/1, Simulation 3D UAV Vehicle/1, TrueCentroidPos/1
  Transpose3/1 -> Simulation 3D UAV Vehicle/2

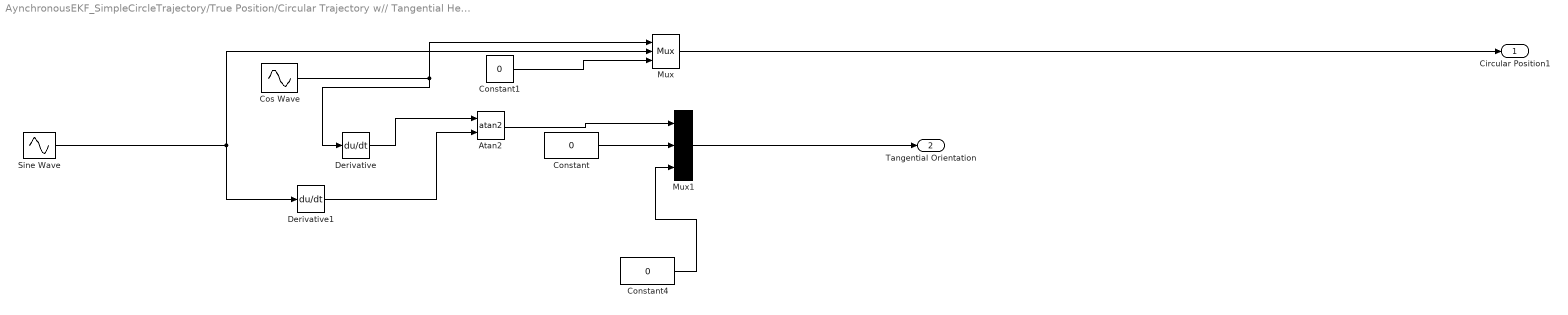
== system AynchronousEKF_SimpleCircleTrajectory/True Position/Circular Trajectory w// Tangential Heading ==
  Atan2 : Trigonometry  Operator=atan2
  Constant : Constant  Value=0  VectorParams1D=off
  Constant1 : Constant  Value=0  VectorParams1D=off
  Constant4 : Constant  Value=0  VectorParams1D=off
  Cos Wave : Sin  Amplitude=radius  Bias=2  Frequency=omega  Phase=pi/2  SampleTime=0  VectorParams1D=off
  Derivative : Derivative
  Derivative1 : Derivative
  Mux : Mux  Inputs=3
  Mux1 : Mux  Inputs=3
  Sine Wave : Sin  Amplitude=radius  Frequency=omega  SampleTime=0  VectorParams1D=off
  Circular Position1 : Outport
  Tangential Orientation : Outport  Port=2
  wires:
  Derivative1/1 -> Atan2/2
  Constant/1 -> Mux1/2
  Constant1/1 -> Mux/3
  Mux1/1 -> Tangential Orientation/1
  Cos Wave/1 -> Mux/1, Derivative/1
  Sine Wave/1 -> Derivative1/1, Mux/2
  Derivative/1 -> Atan2/1
  Atan2/1 -> Mux1/1
  Constant4/1 -> Mux1/3
  Mux/1 -> Circular Position1/1

== matlab function AynchronousEKF_SimpleCircleTrajectory/Cameras/MATLAB Function ==
  data: eulers input; eulerZYX output
function eulerZYX  = swapangles(eulers)
    yaw = eulers(3);
    pitch = eulers(2);
    roll = eulers(1);
    eulerZYX = [yaw, pitch, roll];
end

== matlab function AynchronousEKF_SimpleCircleTrajectory/Colour Segmentation/Colour Segmentation2 ==
  data: cam_LAB input; uv_CamRGBY output; new_frame input
function uv_CamRGBY = coloursegment_UAV(cam_LAB, new_frame)
    if new_frame
        [uv_camR, uv_camG, uv_camB, uv_camY]  = segment_image(cam_LAB);
        uv_CamRGBY = [uv_camR; uv_camG; uv_camB; uv_camY];
    else
        uv_CamRGBY = [NaN, NaN; NaN, NaN; NaN, NaN; NaN, NaN];
    end


end

function [red_uv, green_uv, blue_uv, yellow_uv] = segment_image(imLab)
    a = imLab(:,:,2); %red/green channel
    b = imLab(:,:,3); %blue/yellow channel
    L = imLab(:,:,1);
    % colour thresholds from colour threshold app
    red_mask    = (a > 40) & (b>20);
    red_mask = clean_mask(red_mask);

    green_mask  = (a < -60) & (b > 0);
    green_mask = clean_mask(green_mask);

    blue_mask   =  (b < -40) & (a> 20);
    blue_mask = clean_mask(blue_mask);


    yellow_mask = (b > 50) & (a > -30) & (a< -20) & (L>60);
    yellow_mask = clean_mask(yellow_mask);

    red_uv    = get_centroid(red_mask);
    green_uv  = get_centroid(green_mask);
    blue_uv  = get_centroid(blue_mask);
    yellow_uv  = get_centroid(yellow_mask);
end

function cleaned_mask = clean_mask(mask)
    SE = 20;
    cleaned_mask = bwareaopen(mask, SE);
end

function centroid = get_centroid(mask)
    stats = regionprops(mask, 'Centroid', 'Area');
    if ~isempty(stats)
        areas = zeros(1, numel(stats));
        for i = 1:numel(stats)
            areas(i) = stats(i).Area;
        end
        [~, idx] = max(areas, [], 2); 
        centroid = stats(idx).Centroid;
    else
        centroid = [NaN, NaN];
    end
end

== matlab function AynchronousEKF_SimpleCircleTrajectory/Cameras/MATLAB Function1 ==
  data: eulers input; eulerZYX output
function eulerZYX  = swapangles(eulers)
    yaw = eulers(3);
    pitch = eulers(2);
    roll = eulers(1);
    eulerZYX = [yaw, pitch, roll];
end

== matlab function AynchronousEKF_SimpleCircleTrajectory/Cameras/MATLAB Function2 ==
  data: eulers input; eulerZYX output
function eulerZYX  = swapangles(eulers)
    yaw = eulers(3);
    pitch = eulers(2);
    roll = eulers(1);
    eulerZYX = [yaw, pitch, roll];
end

== matlab function AynchronousEKF_SimpleCircleTrajectory/Cameras/MATLAB Function3 ==
  data: u input; y output
function y = fcn(u)

y = u;

== matlab function AynchronousEKF_SimpleCircleTrajectory/MATLAB Function1 ==
  data: uv input; Position_est output; cams_K input; cams_R input; cams_t input; body_coords input; dt input; Quaternion_est output; x_est_in input; P_est_in input; init_flag_in input; x_est_out output; P_est_out output; init_flag_out output
function [Position_est, Quaternion_est, x_est_out, P_est_out, init_flag_out] = EKF(uv, cams_K, cams_R, cams_t,body_coords, dt, x_est_in, P_est_in, init_flag_in)
    
    %CHANGE THIS WHEN ADDING CAMERAS
    num_cams = 3;
    num_states = 13;
    num_features = 4;
    num_measurements = num_cams*num_features*2; %amount of expected pixels 

    %Initilise to starting positions
    if init_flag_in == 0
        
        % [Px; Py; Pz; Vx; Vy; Vz; q0; qx; qy; qz; omegax; omegay; omegaz]
        Pos_init = [2.6; 0; 0.5];
        V_init = [0; 0.4; 0];        % Initial velocity 
        q_init = [0.707107; 0; 0; 0.707107];
        omega_init = [0; 0.6667 ;0];   % Body omega
        x_est = [Pos_init;V_init;q_init;omega_init];  

        % Initialize state error covariance
        P_est = diag([0.05*ones(1,3), ... 
                     0.005*ones(1,3), ... 
                     0.005*ones(1,4), ... 
                     0.005*ones(1,3)]); 

        init_flag_out = 1; 
        disp('EKF Initialized');
    else
        %Unit delays
        x_est = x_est_in;
        P_est = P_est_in;
        init_flag_out = init_flag_in;
    end
    
    % Process noise Covariance
    Amax = 0.2; % m/s^2, max acceleration
    eA = Amax/sqrt(3)*ones(1,3); %std dev of a uniform distribution
    alpha_max = 0.05; % maximum angular acceleration
    ealpha = alpha_max/sqrt(3)*ones(1,3);  %std dev of a uniform distribution
    Q = diag([eA,ealpha]); %scale by process noise jacobian 
    G = [zeros(3,6); %position: no direct noise
         dt*eye(3), zeros(3); % velocity: acceleration noise
         zeros(4,6); % quaternion: no direct noise
         zeros(3), dt*eye(3)]; %angular velocity: angular acceleration noise 
    Qk = G*Q*G';
    
    %Measurement Noise Covariance 
    pixel_std = 7; %std dev of a uniform distribution 
    R_full = diag((pixel_std^2) * ones(num_measurements, 1));

%Predict
    x_pred = state_transition(x_est,dt); %a priori state

    %State Transition Jacobian
    A_k = compute_StateJacobian(x_pred, dt);

    P_pred = A_k*P_est*A_k' + Qk; 

%Update 
    z = zeros(num_measurements,1); % measurement vector 24x1 for 3 cams
    for cam_idx = 1:num_cams
        for feat_idx = 1:num_features
            meas_idx = (cam_idx -1)*num_features*2 + (feat_idx-1)*2 +1;
            uv_row_start = (cam_idx - 1) * 4 + 1;
            uv_row_end = cam_idx * 4;
            cam_uv = uv(uv_row_start:uv_row_end, :); % 4x2
            z(meas_idx) = cam_uv(feat_idx,1); %u
            z(meas_idx+1) = cam_uv(feat_idx,2); %v
        end
    end

    vis_idx = find(~isnan(z)); 
    z_k = z(vis_idx); 
    [h_k, H_k] = calculate_h_and_H(x_pred, body_coords, cams_K, cams_R, cams_t, num_cams, num_features, vis_idx);
    
    % 
    % if init_flag_in == 1  % Only on second timestep
    %     disp('=== DIAGNOSTIC ===');
    %     disp(['Predicted state P: ', num2str(x_pred(1:3)')]);
    %     disp(['Predicted pixels (h_k): ', num2str(h_k(1:min(8,length(h_k)))')]);
    %     disp(['Measured pixels (z_k): ', num2str(z_k(1:min(8,length(z_k)))')]);
    %     disp(['Num visible: ', num2str(length(vis_idx))]);
    % end

    R_k = R_full(vis_idx, vis_idx);

    y_k = z_k - h_k; %measurement residual 
    
    S_k = H_k*P_pred*H_k' + R_k;
    KG_k = (P_pred*H_k') / S_k;
    x_est = x_pred + KG_k*y_k; %posteriori state update equation

    q_norm = norm(x_est(7:10));
    x_est(7:10) = x_est(7:10) / q_norm;

    I_KH = eye(num_states) - KG_k * H_k; 
    P_est = I_KH * P_pred*I_KH' +KG_k*R_k*KG_k'; %Posteriori process covariance in Joseph form 
    
    %Outputs of centroid position, velocity and body orientation and ang
    %velocity in world frame
    Position_est = x_est(1:3);
    Quaternion_est = x_est(7:10);
    x_est_out = x_est;
    P_est_out = P_est;

    %Debug output - assess perfromance
    disp(['Predicted pixels: ', num2str(h_k')]);
    disp(['Measured pixels: ', num2str(z_k')]);
    disp(['Residual: ', num2str(y_k')]);

    
    % Compute condition number of the measurement Jacobian
    % H_observable = H_k(:, [1:3, 7:10]);  % Only position and quaternion columns
    % H_cond_obs = cond(H_observable);
    % 
    % S_k_temp = H_k * P_pred * H_k' + R_k;
    % S_cond = cond(S_k_temp);
    % 
    % disp(['H_obs cond: ', num2str(H_cond_obs), ' | S cond: ', num2str(S_cond)]);
    % 
    % % Also check if H_k has any content at all
    % H_norm = norm(H_k, 'fro');
    % disp(['H_k norm: ', num2str(H_norm)])
    disp(['Num measurements: ', num2str(length(vis_idx))]);
end

%f(x_pred)
function x_next = state_transition(x_current, dt)
    x_next = zeros(13,1);
    P = x_current(1:3);
    V = x_current(4:6);
    q = x_current(7:10);
    w = x_current(11:13);

    x_next(1:3) = P + V * dt; %position update
    x_next(4:6) = V; %constant velocity assumption
    w_norm = norm(w); %quaternion update
    if w_norm > 0 
        axis = w / w_norm;
        angle = w_norm * dt;
        delta_q = [cos(angle/2); axis*sin(angle/2)];
        x_next(7:10) = quatmultiply(q', delta_q')'; %body frame ang velocity
    else
        x_next(7:10) = q; %No rotation if omega is zero
    end

    q_norm = norm(x_next(7:10));
    if q_norm > 0
        x_next(7:10) = x_next(7:10) / q_norm;
    else
        x_next(7:10) = [1; 0; 0; 0]; 
    end
    x_next(11:13) = w; %constant angular velocity assumption
end

% Calculate the state transition Jacobian
function A_k = compute_StateJacobian(x_pred, dt)
    A_k = eye(13);
    q0 = x_pred(7); 
    qx = x_pred(8); 
    qy = x_pred(9); 
    qz = x_pred(10);
    wx = x_pred(11); 
    wy = x_pred(12); 
    wz = x_pred(13);

    %Position depends on velocity
    A_k(1:3, 4:6) = dt*eye(3);
    %Quaternion depends of prev quat dq/dq
    A_k(7,8:10) = [-dt*wx/2, -dt*wy/2, -dt*wz/2];
    A_k(8,7) = dt*wx/2;
    A_k(8,9) = dt*wz/2;
    A_k(8,10) = -dt*wy/2;
    A_k(9, 7) = dt*wy/2;  
    A_k(9, 8) = -dt*wz/2;  
    A_k(9, 10) = dt*wx/2;
    A_k(10, 7) = dt*wz/2; 
    A_k(10, 8) = dt*wy/2;  
    A_k(10, 9) = -dt*wx/2;
    %Quarternion depends on ang vel. dq/dw
    A_k(7, 11:13) = [-dt*qx/2, -dt*qy/2, -dt*qz/2];
    A_k(8, 11:13) = [dt*q0/2, -dt*qz/2, dt*qy/2];
    A_k(9, 11:13) = [dt*qz/2, dt*q0/2, -dt*qx/2];
    A_k(10, 11:13) = [-dt*qy/2, dt*qx/2, dt*q0/2];
end

% Calculate the measurement function h(x) and the measurement Jacobian H(x)
function [h_k, H_k] = calculate_h_and_H(x_pred, body_coords, cams_K, cams_R, cams_t, num_cams, num_features, vis_idx)
    
    P = x_pred(1:3);     %Position states
    q = x_pred(7:10);    %Quaternion state 
    
    % R_uav = quat2rotm(q'); % Convert quaternion to rotation matrix
    num_meas = num_cams*num_features*2; % 2 cameras × 2 coords (u,v) × features
    
    h_full = zeros(num_meas, 1);
    H_full = zeros(num_meas, 13); 

    for cam_idx = 1:num_cams
        % Row indices for this camera
        row_start = (cam_idx - 1) * 3 + 1;
        row_end = cam_idx * 3;
        
        % Extract camera parameters
        cam_K = cams_K(row_start:row_end, :);    % 3x3
        cam_R = cams_R(row_start:row_end, :);    % 3x3: UE world to UE camera
        cam_t = cams_t(row_start:row_end);       % 3x1: UE world to UE camera
        %transform to openCV cam coord convention from UE world
        % R_ue2cv = [0   1   0;  % openCV x = right, UE y = right 
        %            0   0  -1;  % openCV y = down, UE z = up
        %            1   0   0]; % openCV z = forward, UE x = forward
        

        %MATLAB to intrisic coord transform
        R_rh2cv = [0   -1   0;  % camIntrin x = right, RH y = left
                   0    0  -1;  % camIntrin y = down, RH z = up
                   1    0   0]; % camIntrin z = forwards, RH x= forward

        R_w2cv = R_rh2cv*cam_R;
        t_w2cv = -R_w2cv*cam_t;

        % R_c2w = R_w2cv'; % camera to world (rotation of W wrt C)
        % t_c2w = -R_c2w*t_w2cv; % camera to world pure translation 

        M_ext = [R_w2cv, t_w2cv; 0 0 0 1]; % extrinsics: camera to world 
        M_int = [cam_K, zeros(3,1)]; %intrisics:camera to pixel
        
        for feature_idx = 1:num_features
            %From feature body frame to world frame
            U_bi = body_coords(:, feature_idx); % Body frame coordinates wrt centroid (RGBY order)
            
            point_quat = [0; U_bi(1); U_bi(2); U_bi(3)]; % Convert to pure quaternion and rotate
            q_conj = [q(1); -q(2:4)];
            
            % q * point_quat * q_conj
            temp = quatmultiply(q', point_quat');
            rotated = quatmultiply(temp, q_conj');

            P_world = rotated(2:4)'+P; %Features in world MATLAB RH frame 
            P_cam = M_ext* [P_world; 1]; % homogenous coords of features in camera frame

            UVW = M_int*P_cam; %homog coords camera to image plane
            u = UVW(1)/UVW(3);
            v = UVW(2)/UVW(3);
                    
            meas_idx = (cam_idx - 1) * num_features * 2 + (feature_idx - 1) * 2 + 1;
            u_idx = meas_idx;
            v_idx = meas_idx + 1;
            
            % Store measurements
            h_full(u_idx) = u;
            h_full(v_idx) = v;

            % Compute Measurement Jacobian

            %Transform to camera coordinate frame 
            X_cam = P_cam(1);
            Y_cam = P_cam(2);
            Z_cam = P_cam(3);

            fx = cam_K(1,1);
            fy = cam_K(2,2);

            %Projection Jacobian: dPixel/dCameraCoord
            dpix_dC = [fx/Z_cam, 0, -fx*X_cam/(Z_cam^2); % du/dx,du/dy,du/dz
                         0, fy/Z_cam, -fy*Y_cam/(Z_cam^2)]; %dv/dx,dv/dy,dv/dz
            
            dPc_dPw= R_w2cv;%cam.R;%dCam/dWorld

            dPw_dq = compute_dPw_dq(q, U_bi); %dworld/dquat

            dproj_dPw = dpix_dC * dPc_dPw; % dpix/dCam*dCam/dWorld 

            %Chain rule -> position Jacobian
            dproj_dP = dproj_dPw; % dworld/dPosition = identity matrix 
            
            % Quaternion Jacobian (columns 7-10)
            dproj_dq= dproj_dPw * dPw_dq; % 2x4

            % Fill Jacobian matrix
            H_full(u_idx, 1:3) = dproj_dP(1, :); %Position 
            H_full(u_idx, 7:10) = dproj_dq(1, :); %Quat
            H_full(v_idx, 1:3) = dproj_dP(2, :); %Position
            H_full(v_idx, 7:10) = dproj_dq(2, :); %Quat 
        end
    end
    h_k = h_full(vis_idx);
    H_k = H_full(vis_idx, :);
end

% World point w.r.t. quaternion
function dPw_dq = compute_dPw_dq(q, U_bi)    
    q0 = q(1); 
    qx = q(2); 
    qy = q(3); 
    qz = q(4);
    ux = U_bi(1); %x-coords of body features
    uy = U_bi(2); 
    uz = U_bi(3);
    
    dPw_dq = zeros(3, 4);
    
    %dPw/q0 -> derivate of quat in world frame of body coordinates
    dPw_dq(:,1) = 2*[2*q0*ux + qy*uz - qz*uy;
                     2*q0*uy - qx*uz + qz*ux;
                     2*q0*uz + qx*uy - qy*ux];
    
    %dPw/qx
    dPw_dq(:,2) = 2*[2*qx*ux + qy*uy + qz*uz;
                     qy*ux - q0*uz;
                     qz*ux + q0*uy];
    
    %dPw/qy
    dPw_dq(:,3) = 2*[qx*uy + q0*uz;
                     qx*ux + 2*qy*uy + qz*uz;
                     qz*uy - q0*ux];
    
    %dPw/dqz
    dPw_dq(:,4) = 2*[- q0*uy + qx*uz;
                     q0*ux + qy*uz;
                     qx*ux + qy*uy + 2*qz*uz];
end

== matlab function AynchronousEKF_SimpleCircleTrajectory/Colour Segmentation/Colour Segmentation1 ==
  data: cam_LAB input; new_frame input; uv_CamRGBY output
function uv_CamRGBY = coloursegment_UAV(cam_LAB, new_frame)
    if new_frame
        [uv_camR, uv_camG, uv_camB, uv_camY]  = segment_image(cam_LAB);
        uv_CamRGBY = [uv_camR; uv_camG; uv_camB; uv_camY];
    else
        uv_CamRGBY = [NaN, NaN; NaN, NaN; NaN, NaN; NaN, NaN];
    end


end

function [red_uv, green_uv, blue_uv, yellow_uv] = segment_image(imLab)
    a = imLab(:,:,2); %red/green channel
    b = imLab(:,:,3); %blue/yellow channel
    L = imLab(:,:,1);
    % colour thresholds from colour threshold app
    red_mask    = (a > 40) & (b>20);
    red_mask = clean_mask(red_mask);

    green_mask  = (a < -60) & (b > 0);
    green_mask = clean_mask(green_mask);

    blue_mask   =  (b < -40) & (a> 20);
    blue_mask = clean_mask(blue_mask);


    yellow_mask = (b > 50) & (a > -30) & (a< -20) & (L>60);
    yellow_mask = clean_mask(yellow_mask);

    red_uv    = get_centroid(red_mask);
    green_uv  = get_centroid(green_mask);
    blue_uv  = get_centroid(blue_mask);
    yellow_uv  = get_centroid(yellow_mask);
end

function cleaned_mask = clean_mask(mask)
    SE = 20;
    cleaned_mask = bwareaopen(mask, SE);
end

function centroid = get_centroid(mask)
    stats = regionprops(mask, 'Centroid', 'Area');
    if ~isempty(stats)
        areas = zeros(1, numel(stats));
        for i = 1:numel(stats)
            areas(i) = stats(i).Area;
        end
        [~, idx] = max(areas, [], 2); 
        centroid = stats(idx).Centroid;
    else
        centroid = [NaN, NaN];
    end
end

== matlab function AynchronousEKF_SimpleCircleTrajectory/Colour Segmentation/Colour Segmentation3 ==
  data: cam_LAB input; uv_CamRGBY output; new_frame input
function uv_CamRGBY = coloursegment_UAV(cam_LAB, new_frame)
    if new_frame
        [uv_camR, uv_camG, uv_camB, uv_camY]  = segment_image(cam_LAB);
        uv_CamRGBY = [uv_camR; uv_camG; uv_camB; uv_camY];
    else
        uv_CamRGBY = [NaN, NaN; NaN, NaN; NaN, NaN; NaN, NaN];
    end


end

function [red_uv, green_uv, blue_uv, yellow_uv] = segment_image(imLab)
    a = imLab(:,:,2); %red/green channel
    b = imLab(:,:,3); %blue/yellow channel
    L = imLab(:,:,1);
    % colour thresholds from colour threshold app
    red_mask    = (a > 40) & (b>20);
    red_mask = clean_mask(red_mask);

    green_mask  = (a < -60) & (b > 0);
    green_mask = clean_mask(green_mask);

    blue_mask   =  (b < -40) & (a> 20);
    blue_mask = clean_mask(blue_mask);


    yellow_mask = (b > 50) & (a > -30) & (a< -20) & (L>60);
    yellow_mask = clean_mask(yellow_mask);

    red_uv    = get_centroid(red_mask);
    green_uv  = get_centroid(green_mask);
    blue_uv  = get_centroid(blue_mask);
    yellow_uv  = get_centroid(yellow_mask);
end

function cleaned_mask = clean_mask(mask)
    SE = 20;
    cleaned_mask = bwareaopen(mask, SE);
end

function centroid = get_centroid(mask)
    stats = regionprops(mask, 'Centroid', 'Area');
    if ~isempty(stats)
        areas = zeros(1, numel(stats));
        for i = 1:numel(stats)
            areas(i) = stats(i).Area;
        end
        [~, idx] = max(areas, [], 2); 
        centroid = stats(idx).Centroid;
    else
        centroid = [NaN, NaN];
    end
end
